simulink model "sampleModel1718"  (R2023a)
settings: Solver=VariableStepAuto  StartTime=0.0  StopTime=10.0  RelTol=1e-3
libraries: hdlsllib x7
settings Model: Creator=user1  LastModifiedBy=user1

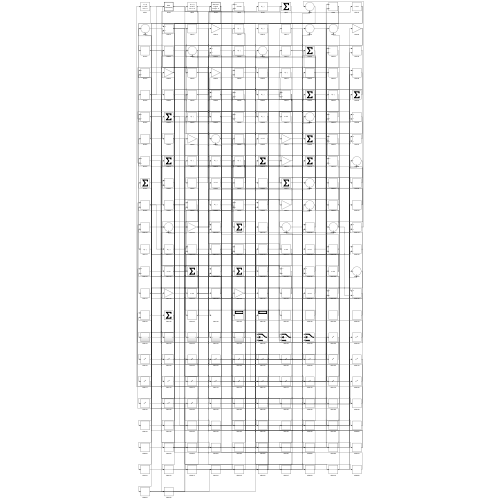
[thumbnail: Simulink's stored preview of the top-level diagram]
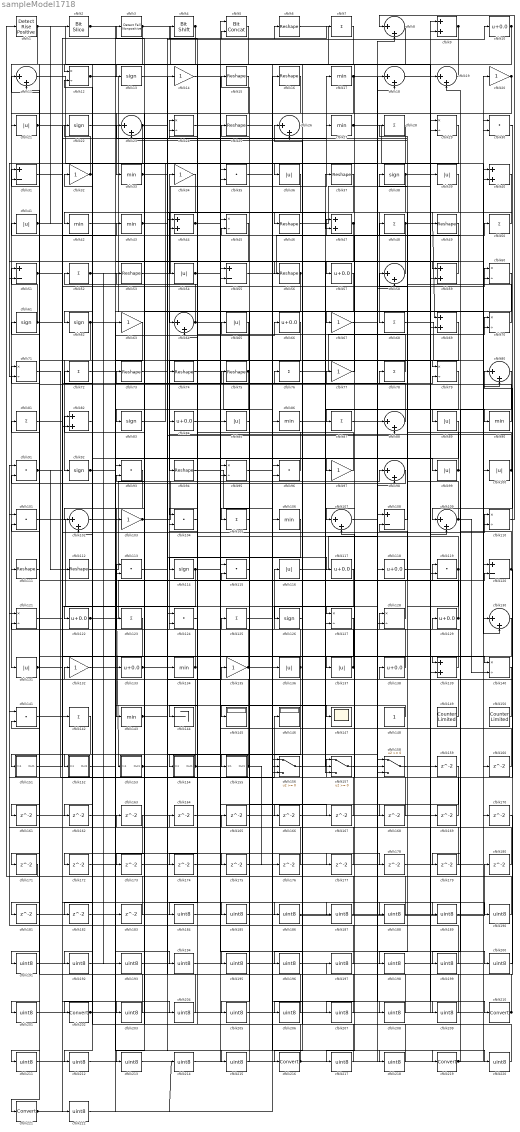
== system sampleModel1718 ==
  cfblk1 : hdlsllib/Logic and Bit Operations/Detect Rise Positive  vinit=0  OutDataTypeStr=boolean
  cfblk{10,57,66,84,117..118,122,129,133,138} (10 alike) : Bias  Bias=0.0  SaturateOnIntegerOverflow=off
  cfblk{21,36,39,41,54,65,85,89,99..100,116,131,136..137} (14 alike) : Abs  SaturateOnIntegerOverflow=off
  cfblk{30,35,91,93,96,101,104,113,115,119,124,141} (12 alike) : DotProduct  OutDataTypeStr=Inherit: Inherit via internal rule
  cfblk{8,11,18..19,23,26,58,64,80,88,98,102,107,109,130} (15 alike) : Sum  Inputs=|++
  cfblk{14,20,32,34,63,67,77,97,103,132,135} (11 alike) : Gain
  cfblk{7,28,48,50,52,68,72,76,78,81,87,105,123,125,142} (15 alike) : Sum  Inputs=+
  cfblk{17,27,33,42..43,86,90,106,134,143} (10 alike) : MinMax
  cfblk{31,51,55,108,120} (5 alike) : Sum  Inputs=+-
  cfblk{12,24,29,45,60,70..71,79,95,110,121,127..128,140} (14 alike) : Product  Inputs=*/  RndMeth=Zero  SaturateOnIntegerOverflow=on
  cfblk{6,15..16,25,37,46,49,53,56,73..75,94,111..112} (15 alike) : Reshape
  cfblk{13,22,38,61..62,83,92,114,126} (9 alike) : Signum
  cfblk{9,40,44,47,59,69,82,139} (8 alike) : Sum
  cfblk144 : Terminator
  cfblk145 : Display
  cfblk146 : Display
  cfblk147 : Scope
  cfblk148 : Constant  SampleTime=-1
  cfblk149 : hdlsllib/Sources/Counter Limited  uplimit=7  tsamp=-1
  cfblk150 : hdlsllib/Sources/Counter Limited  uplimit=7  tsamp=-1
  cfblk151 : Subsystem
      settings: LibrarySourceBlock=|
      | hdlsllib/Ports &
      | Subsystems/Subsystem
  cfblk152 : Subsystem
      settings: LibrarySourceBlock=|
      | hdlsllib/Ports &
      | Subsystems/Subsystem
  cfblk153 : Subsystem
      settings: LibrarySourceBlock=|
      | hdlsllib/Ports &
      | Subsystems/Subsystem
  cfblk154 : Subsystem
      settings: LibrarySourceBlock=|
      | hdlsllib/Ports &
      | Subsystems/Subsystem
  cfblk155 : Subsystem
      settings: LibrarySourceBlock=|
      | hdlsllib/Ports &
      | Subsystems/Subsystem
  cfblk156 : Switch  SaturateOnIntegerOverflow=off  InputSameDT=off
  cfblk157 : Switch  SaturateOnIntegerOverflow=off  InputSameDT=off
  cfblk158 : Switch  SaturateOnIntegerOverflow=off  InputSameDT=off
  cfblk{159..183} (25 alike) : Delay  SampleTime=1
  cfblk{184..201,203..209,211..215,217..218,220,222} (34 alike) : DataTypeConversion  OutDataTypeStr=uint8  SaturateOnIntegerOverflow=off  RndMeth=Floor
  cfblk2 : hdlsllib/Logic and Bit Operations/Bit Slice  lidx=7  ridx=0
  cfblk{202,210,216,219,221} (5 alike) : DataTypeConversion  SaturateOnIntegerOverflow=off  RndMeth=Floor
  cfblk3 : hdlsllib/Logic and Bit Operations/Detect Fall Nonpositive  vinit=0  OutDataTypeStr=boolean
  cfblk4 : hdlsllib/Logic and Bit Operations/Bit Shift  mode=Shift Left Logical  N=0
  cfblk5 : hdlsllib/Logic and Bit Operations/Bit Concat  numInputs=2
  wires:
  cfblk135/1 -> cfblk34/1, cfblk77/1
  cfblk83/1 -> cfblk36/1
  cfblk51/1 -> cfblk7/1, cfblk203/1
  cfblk10/1 -> cfblk131/1, cfblk172/1
  cfblk154/1(Out1) -> cfblk32/1, cfblk178/1
  cfblk78/1 -> cfblk52/1
  cfblk132/1 -> cfblk219/1
  cfblk33/1 -> cfblk46/1, cfblk117/1
  cfblk71/1 -> cfblk146/1
  cfblk63/1 -> cfblk221/1
  cfblk39/1 -> cfblk87/1
  cfblk62/1 -> cfblk92/1, cfblk147/1
  cfblk1/1 -> cfblk111/1, cfblk69/2
  cfblk139/1 -> cfblk116/1
  cfblk65/1 -> cfblk94/1
  cfblk122/1 -> cfblk153/1(In1), cfblk70/2
  cfblk140/1 -> cfblk138/1
  cfblk119/1 -> cfblk64/2, cfblk168/1
  cfblk61/1 -> cfblk51/1, cfblk43/1
  cfblk129/1 -> cfblk71/1, cfblk108/2
  cfblk52/1 -> cfblk64/1, cfblk193/1
  cfblk149/1 -> cfblk82/1
  cfblk53/1 -> cfblk17/1
  cfblk102/1 -> cfblk143/1
  cfblk112/1 -> cfblk85/1
  cfblk47/1 -> cfblk51/2, cfblk83/1, cfblk157/3
  cfblk104/1 -> cfblk24/1
  cfblk60/1 -> cfblk67/1
  cfblk66/1 -> cfblk155/1(In1)
  cfblk25/1 -> cfblk139/1
  cfblk30/1 -> cfblk109/1
  cfblk21/1 -> cfblk134/1, cfblk187/1
  cfblk88/1 -> cfblk3/1
  cfblk44/1 -> cfblk154/1(In1), cfblk99/1
  cfblk48/1 -> cfblk69/1, cfblk157/2, cfblk207/1
  cfblk20/1 -> cfblk21/1, cfblk196/1
  cfblk131/1 -> cfblk110/1, cfblk137/1
  cfblk32/1 -> cfblk62/1, cfblk22/1
  cfblk93/1 -> cfblk202/1
  cfblk8/1 -> cfblk152/1(In1)
  cfblk74/1 -> cfblk136/1
  cfblk82/1 -> cfblk122/1
  cfblk91/1 -> cfblk60/1, cfblk112/1
  cfblk54/1 -> cfblk174/1, cfblk200/1
  cfblk50/1 -> cfblk49/1
  cfblk107/1 -> cfblk50/1
  cfblk12/1 -> cfblk55/2, cfblk60/2, cfblk204/1
  cfblk43/1 -> cfblk14/1, cfblk6/1
  cfblk138/1 -> cfblk128/1
  cfblk118/1 -> cfblk29/1
  cfblk3/1 -> cfblk86/1, cfblk201/1
  cfblk117/1 -> cfblk126/1
  cfblk59/1 -> cfblk57/1
  cfblk151/1(Out1) -> cfblk78/1
  cfblk156/1 -> cfblk37/1
  cfblk5/1 -> cfblk114/1
  cfblk34/1 -> cfblk42/1
  cfblk19/1 -> cfblk13/1
  cfblk70/1 -> cfblk38/1
  cfblk2/1 -> cfblk79/1, cfblk5/2
  cfblk9/1 -> cfblk107/1, cfblk102/2
  cfblk27/1 -> cfblk130/1, cfblk8/2
  cfblk36/1 -> cfblk54/1
  cfblk103/1 -> cfblk5/1, cfblk88/2
  cfblk153/1(Out1) -> cfblk135/1, cfblk120/2
  cfblk133/1 -> cfblk98/1, cfblk27/1, cfblk215/1
  cfblk42/1 -> cfblk110/2
  cfblk75/1 -> cfblk104/1, cfblk123/1
  cfblk143/1 -> cfblk73/1, cfblk156/2
  cfblk96/1 -> cfblk4/1
  cfblk126/1 -> cfblk76/1
  cfblk97/1 -> cfblk65/1
  cfblk155/1(Out1) -> cfblk81/1, cfblk176/1
  cfblk18/1 -> cfblk210/1
  cfblk17/1 -> cfblk158/1, cfblk102/1
  cfblk152/1(Out1) -> cfblk79/2
  cfblk134/1 -> cfblk72/1, cfblk11/2
  cfblk128/1 -> cfblk61/1
  cfblk56/1 -> cfblk105/1, cfblk173/1
  cfblk92/1 -> cfblk66/1, cfblk175/1
  cfblk98/1 -> cfblk91/2
  cfblk157/1 -> cfblk119/1
  cfblk23/1 -> cfblk71/2, cfblk47/2
  cfblk41/1 -> cfblk142/1, cfblk2/1
  cfblk111/1 -> cfblk151/1(In1)
  cfblk28/1 -> cfblk158/2
  cfblk124/1 -> cfblk74/1
  cfblk46/1 -> cfblk9/1
  cfblk38/1 -> cfblk68/1, cfblk140/1
  cfblk116/1 -> cfblk88/1
  cfblk120/1 -> cfblk157/1, cfblk44/2
  cfblk94/1 -> cfblk156/1
  cfblk68/1 -> cfblk130/2
  cfblk136/1 -> cfblk113/1, cfblk181/1
  cfblk87/1 -> cfblk89/1
  cfblk15/1 -> cfblk103/1
  cfblk31/1 -> cfblk127/1
  cfblk100/1 -> cfblk28/1, cfblk84/1
  cfblk72/1 -> cfblk95/2
  cfblk86/1 -> cfblk90/1
  cfblk108/1 -> cfblk58/1
  cfblk101/1 -> cfblk128/2
  cfblk49/1 -> cfblk59/1
  cfblk105/1 -> cfblk25/1
  cfblk114/1 -> cfblk182/1, cfblk188/1
  cfblk81/1 -> cfblk24/2
  cfblk148/1 -> cfblk145/1
  cfblk73/1 -> cfblk10/1
  cfblk85/1 -> cfblk15/1
  cfblk55/1 -> cfblk48/1
  cfblk109/1 -> cfblk41/1, cfblk23/2, cfblk140/2
  cfblk6/1 -> cfblk119/2
  cfblk99/1 -> cfblk23/1, cfblk179/1
  cfblk76/1 -> cfblk70/1
  cfblk77/1 -> cfblk47/1
  cfblk110/1 -> cfblk8/1
  cfblk58/1 -> cfblk56/1
  cfblk24/1 -> cfblk97/1
  cfblk150/1 -> cfblk104/2
  cfblk29/1 -> cfblk82/2
  cfblk26/1 -> cfblk216/1
  cfblk84/1 -> cfblk127/2
  cfblk4/1 -> cfblk12/1, cfblk191/1
  cfblk137/1 -> cfblk31/1, cfblk75/1
  cfblk64/1 -> cfblk53/1, cfblk158/3
  cfblk57/1 -> cfblk133/1
  cfblk16/1 -> cfblk33/1
  cfblk11/1 -> cfblk118/1
  cfblk37/1 -> cfblk144/1
  cfblk90/1 -> cfblk31/2
  cfblk160/1 -> cfblk55/1
  cfblk127/1 -> cfblk161/1
  cfblk161/1 -> cfblk109/2
  cfblk89/1 -> cfblk162/1
  cfblk162/1 -> cfblk139/2
  cfblk164/1 -> cfblk98/2
  cfblk165/1 -> cfblk58/2
  cfblk7/1 -> cfblk166/1
  cfblk166/1 -> cfblk108/1
  cfblk14/1 -> cfblk167/1
  cfblk167/1 -> cfblk95/1
  cfblk168/1 -> cfblk121/1
  cfblk158/1 -> cfblk169/1
  cfblk169/1 -> cfblk107/2
  cfblk123/1 -> cfblk171/1
  cfblk171/1 -> cfblk1/1
  cfblk172/1 -> cfblk19/1
  cfblk173/1 -> cfblk30/2
  cfblk174/1 -> cfblk9/2
  cfblk175/1 -> cfblk29/2
  cfblk176/1 -> cfblk113/2
  cfblk22/1 -> cfblk177/1
  cfblk177/1 -> cfblk11/1
  cfblk178/1 -> cfblk120/1
  cfblk179/1 -> cfblk44/1
  cfblk180/1 -> cfblk91/1
  cfblk181/1 -> cfblk59/2
  cfblk183/1 -> cfblk12/2
  cfblk106/1 -> cfblk184/1
  cfblk184/1 -> cfblk20/1
  cfblk113/1 -> cfblk185/1
  cfblk185/1 -> cfblk106/1
  cfblk141/1 -> cfblk186/1
  cfblk186/1 -> cfblk180/1
  cfblk187/1 -> cfblk141/1
  cfblk188/1 -> cfblk141/2
  cfblk35/1 -> cfblk189/1
  cfblk189/1 -> cfblk129/1
  cfblk13/1 -> cfblk190/1
  cfblk190/1 -> cfblk35/1
  cfblk191/1 -> cfblk35/2
  cfblk40/1 -> cfblk192/1
  cfblk192/1 -> cfblk96/2
  cfblk193/1 -> cfblk40/1
  cfblk182/1 -> cfblk194/1
  cfblk194/1 -> cfblk40/2
  cfblk159/1 -> cfblk195/1
  cfblk195/1 -> cfblk96/1
  cfblk196/1 -> cfblk159/1
  cfblk170/1 -> cfblk197/1
  cfblk197/1 -> cfblk101/1
  cfblk79/1 -> cfblk198/1
  cfblk198/1 -> cfblk170/1
  cfblk80/1 -> cfblk199/1
  cfblk199/1 -> cfblk101/2
  cfblk200/1 -> cfblk80/1
  cfblk201/1 -> cfblk80/2
  cfblk202/1 -> cfblk156/3, cfblk39/1, cfblk218/1
  cfblk203/1 -> cfblk93/1
  cfblk204/1 -> cfblk93/2
  cfblk115/1 -> cfblk205/1
  cfblk205/1 -> cfblk30/1
  cfblk69/1 -> cfblk206/1
  cfblk206/1 -> cfblk115/1
  cfblk207/1 -> cfblk115/2
  cfblk125/1 -> cfblk208/1
  cfblk208/1 -> cfblk124/1
  cfblk67/1 -> cfblk209/1
  cfblk209/1 -> cfblk125/1
  cfblk210/1 -> cfblk124/2, cfblk121/2
  cfblk142/1 -> cfblk211/1
  cfblk211/1 -> cfblk18/1
  cfblk163/1 -> cfblk212/1
  cfblk212/1 -> cfblk18/2
  cfblk45/1 -> cfblk213/1
  cfblk213/1 -> cfblk100/1
  cfblk214/1 -> cfblk45/1
  cfblk215/1 -> cfblk45/2
  cfblk216/1 -> cfblk165/1, cfblk164/1, cfblk163/1
  cfblk130/1 -> cfblk217/1
  cfblk217/1 -> cfblk26/1
  cfblk218/1 -> cfblk26/2
  cfblk219/1 -> cfblk160/1, cfblk19/2
  cfblk95/1 -> cfblk220/1
  cfblk220/1 -> cfblk132/1
  cfblk221/1 -> cfblk214/1, cfblk183/1, cfblk16/1
  cfblk121/1 -> cfblk222/1
  cfblk222/1 -> cfblk63/1

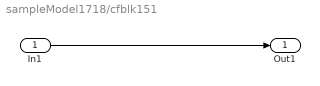
== system sampleModel1718/cfblk151 ==
  In1 : Inport
  Out1 : Outport
  wires:
  In1/1 -> Out1/1

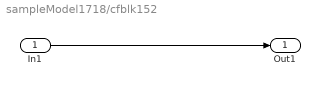
== system sampleModel1718/cfblk152 ==
  In1 : Inport
  Out1 : Outport
  wires:
  In1/1 -> Out1/1

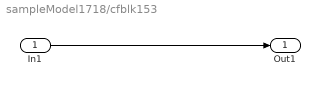
== system sampleModel1718/cfblk153 ==
  In1 : Inport
  Out1 : Outport
  wires:
  In1/1 -> Out1/1

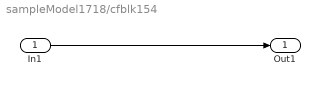
== system sampleModel1718/cfblk154 ==
  In1 : Inport
  Out1 : Outport
  wires:
  In1/1 -> Out1/1

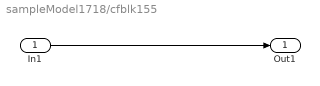
== system sampleModel1718/cfblk155 ==
  In1 : Inport
  Out1 : Outport
  wires:
  In1/1 -> Out1/1
